simulink subsystem "DAC_SubSystem"  (R2020b)
settings: Solver=VariableStepAuto  StartTime=0.0  StopTime=10.0  RelTol=1e-3
values from neighbouring files (symbols this model uses):
  Ts = 0.001    [loadParNominalHubBeam.m]
undefined symbols (not defined in the file or in its folder): daq
settings Model: Creator=umberto  LastModifiedBy=umberto

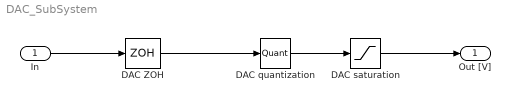
== system DAC_SubSystem ==
  In : Inport
  DAC ZOH : ZeroOrderHold  SampleTime=Ts
  DAC quantization : Quantizer  QuantizationInterval=daq.dac.q
  DAC saturation : Saturate  UpperLimit=daq.dac.fs  LowerLimit=-daq.dac.fs
  Out [V] : Outport
  wires:
  In/1 -> DAC ZOH/1
  DAC ZOH/1 -> DAC quantization/1
  DAC quantization/1 -> DAC saturation/1
  DAC saturation/1 -> Out [V]/1
